simulink model "Linearize_Bare_Airframe"  (R2022a)
settings: Solver=VariableStepAuto  StartTime=0.0  StopTime=10.0  RelTol=1e-3
undefined symbols (not defined in the file): Aactuator, ac, AeroCoeff, EngineTable, F, fs, ft, g, hground, IC, kg, LandingGear, Light, m, MIL, s, Sensor, slug, state0, WMM2020
libraries: aerolibconvert2 x15, simulink x4, aerolibatmos2 x3, aerolibwind2 x3, sharedutil x3, aerolibbdyn x3, aerolibgravity2 x2, sharedtransform x1
(part 1 of 4)
settings Model: Creator=user  LastModifiedBy=user

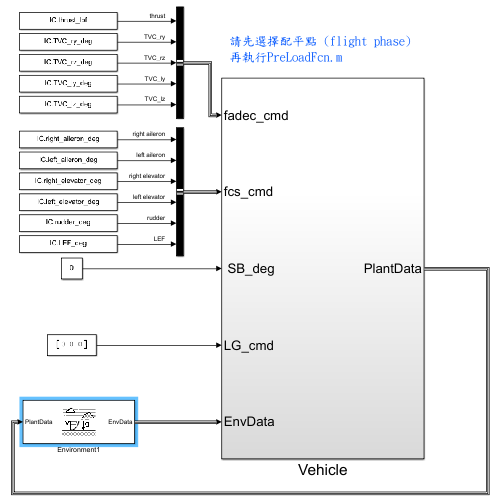
[thumbnail: Simulink's stored preview of the top-level diagram]
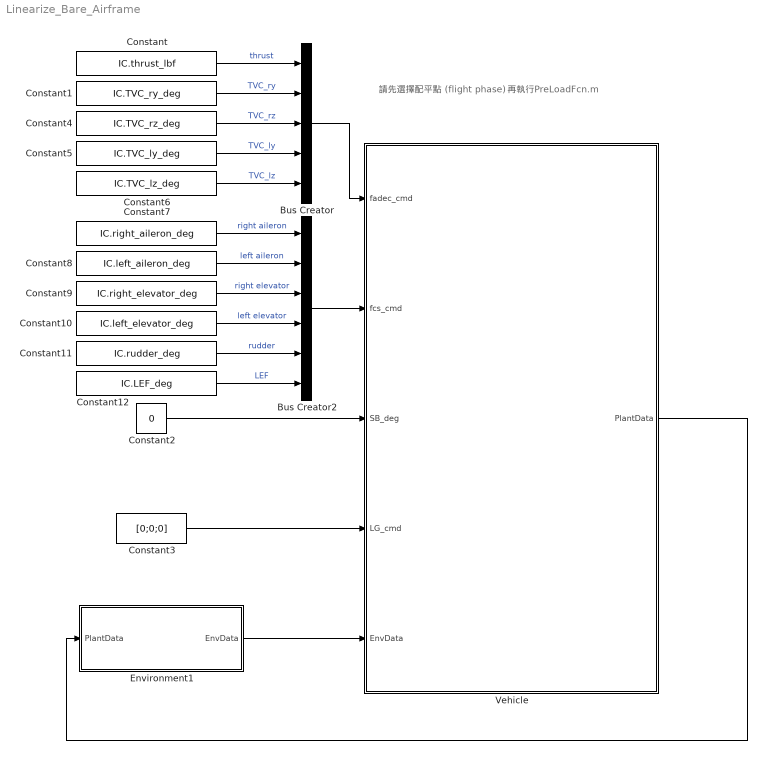
== system Linearize_Bare_Airframe ==
  note: 請先選擇配平點 (flight phase)
      | 再執行PreLoadFcn.m
  Bus Creator : BusCreator  Inputs=5
  Bus Creator2 : BusCreator  Inputs=6
  Constant : Constant  Value=IC.thrust_lbf
  Constant1 : Constant  Value=IC.TVC_ry_deg
  Constant10 : Constant  Value=IC.left_elevator_deg
  Constant11 : Constant  Value=IC.rudder_deg
  Constant12 : Constant  Value=IC.LEF_deg
  Constant2 : Constant  Value=0
  Constant3 : Constant  Value=[0;0;0]
  Constant4 : Constant  Value=IC.TVC_rz_deg
  Constant5 : Constant  Value=IC.TVC_ly_deg
  Constant6 : Constant  Value=IC.TVC_lz_deg
  Constant7 : Constant  Value=IC.right_aileron_deg
  Constant8 : Constant  Value=IC.left_aileron_deg
  Constant9 : Constant  Value=IC.right_elevator_deg
  Environment1 : Subsystem
      mask Display:
      | image('aeroenvironment.bmp','center')
      | % 左側 "Icon transparency" 欄位已選擇 "Opaque with ports"，所以埠名稱會自動顯示，不用再宣告
      | % port_label('input',1,'PlantData')
      | % port_label('output',1,'EnvData')
  Vehicle : Subsystem
  wires:
  Constant3/1 -> Vehicle/4(LG_cmd)
  Constant2/1 -> Vehicle/3(" SB_deg")
  Environment1/1(EnvData) -> Vehicle/5(EnvData)
  Vehicle/1(PlantData) -> Environment1/1(PlantData)
  Constant11/1 -> Bus Creator2/5  "rudder"
  Constant5/1 -> Bus Creator/4  "TVC_ly"
  Constant12/1 -> Bus Creator2/6  "LEF"
  Bus Creator2/1 -> Vehicle/2(fcs_cmd)
  Constant1/1 -> Bus Creator/2  "TVC_ry"
  Constant8/1 -> Bus Creator2/2  "left aileron"
  Constant6/1 -> Bus Creator/5  "TVC_lz"
  Constant/1 -> Bus Creator/1  "thrust"
  Bus Creator/1 -> Vehicle/1(fadec_cmd)
  Constant10/1 -> Bus Creator2/4  "left elevator"
  Constant7/1 -> Bus Creator2/1  "right aileron"
  Constant4/1 -> Bus Creator/3  "TVC_rz"
  Constant9/1 -> Bus Creator2/3  "right elevator"

== system Linearize_Bare_Airframe/Environment1 ==
  note: p, q, r
  note: u, v, w
  note: Wind Models
  note: Atmosphere Model
  note: Altitude must be less than 20000 m (approximately 65620 feet).
  note: 建模注意： EnvData Bus 內要指定公制/英制單位
  note: Magnetic Field
  note: Gravity Model
  note: TODO: 改用這個現成模塊...
      | 但NDI控制器內的重力g是用常數，將產生誤差...
  note: TODO: 改用這個現成模塊...
      | 參考MATLAB Help範例 Quadcopter Project
  note: TODO: 改用現成模塊，改成英制。
      | NDI控制器，不會產生誤差，因為可轉成C程式碼
  note: TODO: 參考MATLAB Help範例 HL-20
      | 將風速效應加到氣動力攻角、側滑角、qbar、Mach、V
  In Bus Element3 : Inport  PortName=PlantData  Element=Vt
  In Bus Element4 : Inport  PortName=PlantData  Element=Vt
  In Bus Element : Inport  PortName=PlantData  Element=DCM_be
  COESA Atmosphere Model : aerolibatmos2/COESA Atmosphere Model  Commented=on  units=English (Velocity in ft/s)  spec=1976 COESA-extended U.S. Standard Atmosphere  model=Profile  profile_var=High temperature  profile_percent=1%  profile_alt=5 km (16404 ft)  envelope_var=High temperature  envelope_percent=1%  action=Warning
  Constant1 : Constant  Value=IC.alt
  Constant12 : Constant  Value=IC.alt
  Constant2 : Constant  Value=IC.Vt
  Density Conversion : aerolibconvert2/Density Conversion  IU=kg/m^3  OU=slug/ft^3
      settings: SourceProductBaseCode=AE
  Discrete Wind Gust Model : aerolibwind2/Discrete Wind Gust Model  Commented=on  units=English (Velocity in ft/s)  Gx=on  Gy=on  Gz=on  t_0=5  d_m=[120 120 80]  v_m=[3.5 3.5 3.0]
  Dryden Wind Turbulence Model (Continuous (+q +r)) : aerolibwind2/Dryden Wind Turbulence Model  (Continuous (+q -r))  Commented=on  units=English (Velocity in ft/s)  spec=MIL-F-8785C  model=Continuous Dryden (+q +r)  W20=15  Wdeg=0  TurbProb=10^-2 - Light  L_high=533.4  Wingspan=10  ts=0.1  Seed=[23341 23342 23343 23344]  T_on=on
  Dynamic Pressure : Subsystem
  Geoid Height : aerolibgravity2/Geoid Height  Commented=on  units=English  gtype=EGM96  datafile='geoidegm96grid'  dtype=double  action=Warning
      settings: AttributesFormatString=EGM2008 Geoid Data Unavailable  SourceProductBaseCode=AE
  ISA Atmosphere Model : aerolibatmos2/ISA Atmosphere Model  Commented=on  custom=off  g=9.80665  gamma=1.4  R=287.0531  L=0.0065  h_trop=11000  h_strat=20000  rho0=1.225  P0=101325  T0=288.15  h0=0
  "ISP " : Subsystem
  Length Conversion : aerolibconvert2/Length Conversion  IU=ft  OU=m
  Mach Number : Subsystem
  Magnetic Field : Constant  Value=[0 0 0]
  Manual Switch : ManualSwitch
  Manual Switch1 : ManualSwitch  CurrentSetting=0
  Pressure Altitude : aerolibatmos2/Pressure Altitude  Commented=on  units=English  action=Warning
      settings: SourceProductBaseCode=AE
  Sum : Sum  Commented=on  Inputs=+++
  Velocity Conversion : aerolibconvert2/Velocity Conversion  IU=m/s  OU=ft/s
  "WGS84 Gravity Model  " : GravityWGS84  Commented=on  units=English
  Wind Shear Model : aerolibwind2/Wind Shear Model  Commented=on  units=English (Velocity in ft/s)  phase=Category C - Terminal Flight Phase  W_20=15  Wdeg=0
  World Magnetic Model : aerolibgravity2/World Magnetic Model  Commented=on  model=WMM2020 (2020-2025)  customFile='WMM2020.COF'  units=English  time_in=on  month=January  day=1  year=2020  action=Error  h_out=off  dec_out=off  inc_out=off  ti_out=off
      settings: SourceProductBaseCode=AE
  gravity (ft/s^2) : Constant  Value=g
  hground (ft) : Constant  Value=hground
  no wind : Constant  Value=[0 0 0]
  no wind1 : Constant  Value=[0 0 0]
  r2d1 : Gain  Commented=on  Gain=-1  SaturateOnIntegerOverflow=on  OutDataTypeStr=Inherit: Same as input  ParamDataTypeStr=Inherit: Same as input
  r2d2 : Gain  Gain=-1  SaturateOnIntegerOverflow=on  OutDataTypeStr=Inherit: Same as input  ParamDataTypeStr=Inherit: Same as input
  Out Bus Element : Outport  PortName=EnvData  Element=Pressure
  Out Bus Element1 : Outport  PortName=EnvData  Element=AirDensity
  Out Bus Element2 : Outport  PortName=EnvData  Element=qbar
  Out Bus Element3 : Outport  PortName=EnvData  Element=Mach
  Out Bus Element4 : Outport  PortName=EnvData  Element=g
  Out Bus Element5 : Outport  PortName=EnvData  Element=hground
  Out Bus Element6 : Outport  PortName=EnvData  Element=MagneticField_NED
  Out Bus Element7 : Outport  PortName=EnvData  Element=AirTemperature_K
  Out Bus Element8 : Outport  PortName=EnvData  Element=SoundSpeed_ms
  Out Bus Element9 : Outport  PortName=EnvData  Element=WindVelocity
  Out Bus Element10 : Outport  PortName=EnvData  Element=WindAngularRates
  wires:
  "ISP "/1(T (K)) -> Out Bus Element7/1
  "ISP "/3(P (HPa)) -> Out Bus Element/1
  "ISP "/4(rho (kg/m^3)) -> Density Conversion/1, Out Bus Element1/1
  hground (ft)/1 -> Out Bus Element5/1
  gravity (ft/s^2)/1 -> Out Bus Element4/1  "Gravity_NED"
  Magnetic Field/1 -> Out Bus Element6/1  "MagneticField_NED"
  Constant12/1 -> r2d2/1
  r2d2/1 -> Length Conversion/1  "h(ft)"
  Length Conversion/1 -> "ISP "/1(h(m))
  "ISP "/2(a (m/s)) -> Out Bus Element8/1, Velocity Conversion/1
  Mach Number/1(Mach) -> Out Bus Element3/1
  Dynamic Pressure/1(qbar) -> Out Bus Element2/1
  Density Conversion/1 -> Dynamic Pressure/2(rho)
  In Bus Element3/1 -> Dynamic Pressure/1(Vt)  "Vt (ft/s)"
  In Bus Element4/1 -> Mach Number/1(Vt)  "Vt (ft/s)"
  Velocity Conversion/1 -> Mach Number/2(a)
  COESA Atmosphere Model/3 -> Pressure Altitude/1
  r2d1/1 -> Dryden Wind Turbulence Model (Continuous (+q +r))/1, Wind Shear Model/1  "h(ft)"
  Constant1/1 -> r2d1/1
  Constant2/1 -> Discrete Wind Gust Model/1, Dryden Wind Turbulence Model (Continuous (+q +r))/2  "Vt (ft/s)"
  In Bus Element/1 -> Wind Shear Model/2, Dryden Wind Turbulence Model (Continuous (+q +r))/3
  Dryden Wind Turbulence Model (Continuous (+q +r))/1 -> Sum/2
  Discrete Wind Gust Model/1 -> Sum/3
  Wind Shear Model/1 -> Sum/1
  Dryden Wind Turbulence Model (Continuous (+q +r))/2 -> Manual Switch1/1  "WindAngularRates"
  Sum/1 -> Manual Switch/2  "WindVelocity"
  Manual Switch/1 -> Out Bus Element9/1
  no wind/1 -> Manual Switch/1
  Manual Switch1/1 -> Out Bus Element10/1
  no wind1/1 -> Manual Switch1/2

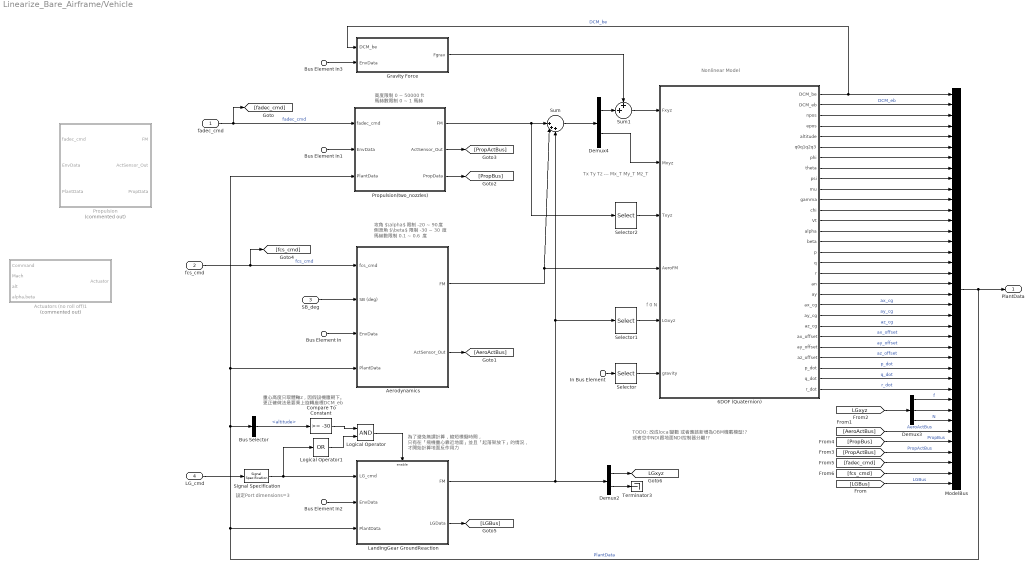
== system Linearize_Bare_Airframe/Vehicle ==
  note: 重心高度只取體軸z，因假設機腹朝下。
      | 更正確做法是要乘上旋轉座標DCM_eb
  note: 為了避免無謂計算，縮短模擬時間，
      | 只有在「飛機重心靠近地面」並且「起落架放下」的情況，
      | 才開始計算地面反作用力
  note: 設定Port dimensions=3
  note: 攻角 $\alpha$ 限制 -20 ~ 90度
      | 側滑角 $\beta$ 限制 -30 ~ 30 度
      | 馬赫數限制 0.1 ~ 0.6 度
  note: Tx
      | Ty
      | Tz
      | ---
      | Mx_T
      | My_T
      | Mz_T
  note: 高度限制 0 ~ 50000 ft
      | 馬赫數限制 0 ~ 1 馬赫
  note: f
      | 0
      | N
  note: TODO: 改成local變數
      | 或者應該新增為OBM機載模型!?
      | 或者空中NDI跟地面NDI控制器分離!?
  note: Nonlinear Model
  fadec_cmd : Inport
  fcs_cmd : Inport  Port=2
  " SB_deg" : Inport  Port=3
  LG_cmd : Inport  Port=4
  Bus Element In{,1..3} (4 alike) : Inport  Port=5  PortName=EnvData
  In Bus Element : Inport  Port=5  PortName=EnvData  Element=g
  6DOF (Quaternion) : Subsystem
  Actuators (no roll off)1 : Subsystem  Commented=on
  Aerodynamics : Subsystem
  Bus Selector : BusSelector  OutputSignals=altitude
  Compare To Constant : simulink/Logic and Bit Operations/Compare To Constant  relop=>=  const=-30  OutDataTypeStr=boolean
  Demux2 : Demux  Outputs=[3, 3]
  Demux3 : Demux  Outputs=3
  Demux4 : Demux  Outputs=[3, 3]
  Gravity Force : Subsystem
  LandingGear GroundReaction : Subsystem
  Logical Operator : Logic  AllPortsSameDT=off  OutDataTypeStr=boolean
  Logical Operator1 : Logic  Operator=OR  Inputs=1  AllPortsSameDT=off  OutDataTypeStr=boolean
  ModelBus : BusCreator  Inputs=38
  Propulsion : Subsystem  Commented=on
  Propulsion(two_nozzles) : Subsystem
  Selector : Selector  InputPortWidth=3  IndexOptions=Index vector (dialog)  Indices=3  OutputSizes=1
  Selector1 : Selector  InputPortWidth=6  IndexOptions=Index vector (dialog)  Indices=[1 2 3]  OutputSizes=1
  Selector2 : Selector  InputPortWidth=6  IndexOptions=Index vector (dialog)  Indices=[1 2 3]  OutputSizes=1
  Signal Specification : SignalSpecification  Dimensions=3
  Sum : Sum  Inputs=||+++
  Sum1 : Sum  Inputs=++|
  Terminator3 : Terminator
  PlantData : Outport
  tag scope: LGxyz=global
  wires:
  " SB_deg"/1 -> Aerodynamics/2(" SB (deg)")
  Aerodynamics/1(FM) -> Sum/2, 6DOF (Quaternion)/4(AeroFM)
  Aerodynamics/2(ActSensor_Out) -> [AeroActBus]
  Propulsion(two_nozzles)/1(FM) -> Selector2/1, Sum/1
  fcs_cmd/1 -> Aerodynamics/1(fcs_cmd), [fcs_cmd]  "fcs_cmd"
  fadec_cmd/1 -> Propulsion(two_nozzles)/1(fadec_cmd), [fadec_cmd]  "fadec_cmd"
  Propulsion(two_nozzles)/2(ActSensor_Out) -> [PropActBus]
  Propulsion(two_nozzles)/3(PropData) -> [PropBus]
  Sum/1 -> Demux4/1
  Sum1/1 -> 6DOF (Quaternion)/1(Fxyz)
  Bus Element In/1 -> Aerodynamics/3(EnvData)
  Bus Element In1/1 -> Propulsion(two_nozzles)/2(EnvData)
  LandingGear GroundReaction/1(FM) -> Demux2/1, Sum/3, Selector1/1
  Selector1/1 -> 6DOF (Quaternion)/5(LGxyz)
  Demux2/1 -> [LGxyz]
  Demux2/2 -> Terminator3/1
  Signal Specification/1 -> Logical Operator1/1, LandingGear GroundReaction/1(LG_cmd)
  LandingGear GroundReaction/2(LGData) -> [LGBus]
  Logical Operator/1 -> LandingGear GroundReaction/Enable
  Compare To Constant/1 -> Logical Operator/1
  Bus Selector/1 -> Compare To Constant/1  "<altitude>"
  Logical Operator1/1 -> Logical Operator/2
  LG_cmd/1 -> Signal Specification/1
  Gravity Force/1(Fgrav) -> Sum1/1
  Demux4/1 -> Sum1/2
  Bus Element In3/1 -> Gravity Force/2(EnvData)
  Bus Element In2/1 -> LandingGear GroundReaction/2(EnvData)
  In Bus Element/1 -> Selector/1
  [PropActBus] -> ModelBus/35  "PropActBus"
  Demux3/2 -> ModelBus/31
  6DOF (Quaternion)/22(ay_cg) -> ModelBus/22  "ay_cg"
  Demux3/3 -> ModelBus/32  "N"
  Demux3/1 -> ModelBus/30  "f"
  6DOF (Quaternion)/2(DCM_eb) -> ModelBus/2  "DCM_eb"
  6DOF (Quaternion)/18(r) -> ModelBus/18
  6DOF (Quaternion)/8(theta) -> ModelBus/8
  [fadec_cmd] -> ModelBus/36
  6DOF (Quaternion)/21(ax_cg) -> ModelBus/21  "ax_cg"
  [LGBus] -> ModelBus/38  "LGBus"
  6DOF (Quaternion)/3(npos) -> ModelBus/3
  6DOF (Quaternion)/10(mu) -> ModelBus/10
  [fcs_cmd] -> ModelBus/37
  [AeroActBus] -> ModelBus/33  "AeroActBus"
  6DOF (Quaternion)/16(p) -> ModelBus/16
  6DOF (Quaternion)/17(q) -> ModelBus/17
  6DOF (Quaternion)/13(Vt) -> ModelBus/13
  6DOF (Quaternion)/29(r_dot) -> ModelBus/29  "r_dot"
  6DOF (Quaternion)/24(ax_offset) -> ModelBus/24  "ax_offset"
  6DOF (Quaternion)/28(q_dot) -> ModelBus/28  "q_dot"
  6DOF (Quaternion)/19(an) -> ModelBus/19
  6DOF (Quaternion)/20(ay) -> ModelBus/20
  6DOF (Quaternion)/6(q0q1q2q3) -> ModelBus/6
  6DOF (Quaternion)/11(gamma) -> ModelBus/11
  6DOF (Quaternion)/27(p_dot) -> ModelBus/27  "p_dot"
  6DOF (Quaternion)/9(psi) -> ModelBus/9
  6DOF (Quaternion)/5(altitude) -> ModelBus/5
  6DOF (Quaternion)/7(phi) -> ModelBus/7
  6DOF (Quaternion)/14(alpha) -> ModelBus/14
  6DOF (Quaternion)/4(epos) -> ModelBus/4
  6DOF (Quaternion)/15(beta) -> ModelBus/15
  6DOF (Quaternion)/1(DCM_be) -> Gravity Force/1(DCM_be), ModelBus/1  "DCM_be"
  6DOF (Quaternion)/23(az_cg) -> ModelBus/23  "az_cg"
  [LGxyz] -> Demux3/1
  ModelBus/1 -> PlantData/1, LandingGear GroundReaction/3(PlantData), Bus Selector/1, Propulsion(two_nozzles)/3(PlantData), Aerodynamics/4(PlantData)  "PlantData"
  6DOF (Quaternion)/25(ay_offset) -> ModelBus/25  "ay_offset"
  6DOF (Quaternion)/12(chi) -> ModelBus/12
  [PropBus] -> ModelBus/34  "PropBus"
  6DOF (Quaternion)/26(az_offset) -> ModelBus/26  "az_offset"
  Demux4/2 -> 6DOF (Quaternion)/2(Mxyz)
  Selector2/1 -> 6DOF (Quaternion)/3(Txyz)
  Selector/1 -> 6DOF (Quaternion)/6(gravity)

== system Linearize_Bare_Airframe/Environment1/Dynamic Pressure ==
  Vt : Inport
  rho : Inport  Port=2
  1/2rhoV^2 : Gain  Gain=1/2  SaturateOnIntegerOverflow=on  OutDataTypeStr=Inherit: Same as input  ParamDataTypeStr=Inherit: Same as input
  Product2 : Product  InputSameDT=on  SaturateOnIntegerOverflow=on  OutDataTypeStr=Inherit: Same as first input
  Square : Math  Operator=square  SignedPower=on
  qbar : Outport
  wires:
  rho/1 -> Product2/2
  Square/1 -> Product2/1
  1/2rhoV^2/1 -> qbar/1
  Product2/1 -> 1/2rhoV^2/1
  Vt/1 -> Square/1

== system Linearize_Bare_Airframe/Environment1/ISP  ==
  note: 1 T
      | 2 a (Speed of sound)
      | 3 P
      | 4 rho
      | 5 g
      | 6 mu (Coefficient of viscosity)
  h(m) : Inport
  Demux : Demux  Outputs=[1,1,1,1,1,1]
      settings: DisplayOption=none
  MATLAB Function : MATLAB Function  TreatAsAtomicUnit=on
  end8 : Terminator
  end9 : Terminator
  T (K) : Outport  VectorParamsAs1DForOutWhenUnconnected=off
  a (m/s) : Outport  Port=2  VectorParamsAs1DForOutWhenUnconnected=off
  P (HPa) : Outport  Port=3  VectorParamsAs1DForOutWhenUnconnected=off
  rho (kg/m^3) : Outport  Port=4  VectorParamsAs1DForOutWhenUnconnected=off
  wires:
  MATLAB Function/1(ISP_output) -> Demux/1
  h(m)/1 -> MATLAB Function/1(h)
  Demux/4 -> rho (kg/m^3)/1  "rho(kg/m^3)"
  Demux/2 -> a (m/s)/1  "a(m/s)"
  Demux/1 -> T (K)/1  "T(K)"
  Demux/5 -> end8/1  "g (m/s^2)"
  Demux/6 -> end9/1  "mu"
  Demux/3 -> P (HPa)/1  "P(Pa)"

== system Linearize_Bare_Airframe/Environment1/Mach Number ==
  Vt : Inport
  a : Inport  Port=2
  Product1 : Product  Inputs=*/  InputSameDT=on  SaturateOnIntegerOverflow=on  OutDataTypeStr=Inherit: Same as first input
  Mach : Outport  Unit=1  VectorParamsAs1DForOutWhenUnconnected=off
  wires:
  Vt/1 -> Product1/1
  a/1 -> Product1/2
  Product1/1 -> Mach/1

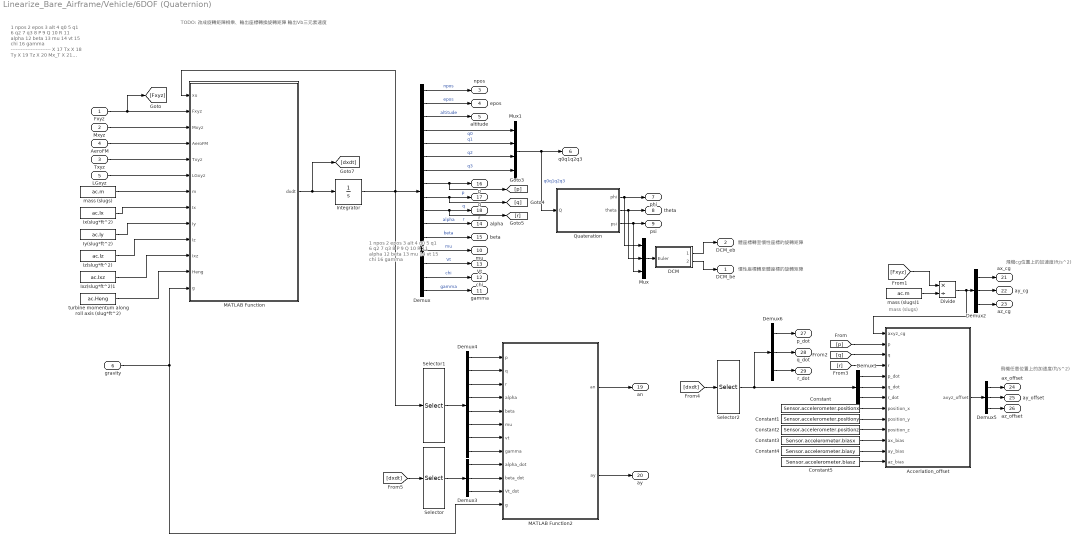
== system Linearize_Bare_Airframe/Vehicle/6DOF (Quaternion) ==
  note: TODO: 改成旋轉矩陣相乘、輸出座標轉換旋轉矩陣
      | 輸出Vb三元素速度
  note: 1 npos
      | 2 epos
      | 3 alt
      | 4 q0
      | 5 q1
      | 6 q2
      | 7 q3
      | 8 P
      | 9 Q
      | 10 R
      | 11 alpha
      | 12 beta
      | 13 mu
      | 14 vt
      | 15 chi
      | 16 gamma
      | ------------------------
      | X 17 Tx
      | X 18 Ty
      | X 19 Tz
      | X 20 Mx_T
      | X 21 My_T
      | X 22 Mz_T
      | X 23 T
      | --------------------
      | X 24 ele
      | X 25 ail
      | X 26 rud
      | -------------------
      | X 27 delta_z
      | X 28 delta_y
      | -----------------
      | X 29 qbar
      | -----------------
      | X 30 CXT
      | X 31 CYT
      | X 32 CZT
      | X 33 CLT
      | X 34 CMT
      | X 35 CNT
      | -----------------
      | X 36 lef
  note: 1 npos
      | 2 epos
      | 3 alt
      | 4 q0
      | 5 q1
      | 6 q2
      | 7 q3
      | 8 P
      | 9 Q
      | 10 R
      | 11 alpha
      | 12 beta
      | 13 mu
      | 14 vt
      | 15 chi
      | 16 gamma
  note: 慣性座標轉至體座標的旋轉矩陣
  note: 體座標轉至慣性座標的旋轉矩陣
  note: mass (slugs)
  note: 飛機cg位置上的加速度(ft/s^2)
  note: 飛機任意位置上的加速度(ft/s^2)
  Fxyz : Inport
  Mxyz : Inport  Port=2
  Txyz : Inport  Port=3
  AeroFM : Inport  Port=4
  LGxyz : Inport  Port=5
  gravity : Inport  Port=6
  Accerlation_offset : Subsystem
  Constant : Constant  Value=Sensor.accelerometer.positionx
  Constant1 : Constant  Value=Sensor.accelerometer.positiony
  Constant2 : Constant  Value=Sensor.accelerometer.positionz
  Constant3 : Constant  Value=Sensor.accelerometer.biasx
  Constant4 : Constant  Value=Sensor.accelerometer.biasy
  Constant5 : Constant  Value=Sensor.accelerometer.biasz
  DCM : Subsystem
  Demux : Demux  Outputs=16
      settings: DisplayOption=none
  Demux{1..3,5..6} (5 alike) : Demux  Outputs=3
  Demux4 : Demux  Outputs=8
  Divide : Product  Inputs=*/
  Integrator : Integrator  InitialCondition=state0  ContinuousStateAttributes={'npos', 'epos', 'alt', 'q0', 'q1', 'q2', 'q3', 'P', 'Q', 'R', 'alpha', 'beta', 'mu', 'vt', 'chi', 'gamma'}
  Ix(slug*ft^2) : Constant  Value=ac.Ix
  Ixz(slug*ft^2)1 : Constant  Value=ac.Ixz
  Iy(slug*ft^2) : Constant  Value=ac.Iy
  Iz(slug*ft^2) : Constant  Value=ac.Iz
  MATLAB Function : MATLAB Function  TreatAsAtomicUnit=on
  MATLAB Function2 : MATLAB Function  TreatAsAtomicUnit=on
  Mux : Mux  Inputs=3
  Mux1 : Mux  Inputs=[1,1,1,1]
  Quateration : MATLAB Function  TreatAsAtomicUnit=on
  Selector : Selector  InputPortWidth=16  IndexOptions=Index vector (dialog)  Indices=[11 12 14]  OutputSizes=3
  Selector1 : Selector  InputPortWidth=16  IndexOptions=Index vector (dialog)  Indices=[8:14 16]  OutputSizes=3
  Selector2 : Selector  InputPortWidth=16  IndexOptions=Index vector (dialog)  Indices=[8 9 10]  OutputSizes=3
  mass (slugs) : Constant  Value=ac.m
  mass (slugs)1 : Constant  Value=ac.m
  turbine momentum along roll axis (slug*ft^2) : Constant  Value=ac.Heng
  DCM_be : Outport
  DCM_eb : Outport  Port=2
  npos : Outport  Port=3  VectorParamsAs1DForOutWhenUnconnected=off
  epos : Outport  Port=4  VectorParamsAs1DForOutWhenUnconnected=off
  altitude : Outport  Port=5  VectorParamsAs1DForOutWhenUnconnected=off
  q0q1q2q3 : Outport  Port=6
  phi : Outport  Port=7  VectorParamsAs1DForOutWhenUnconnected=off
  theta : Outport  Port=8  VectorParamsAs1DForOutWhenUnconnected=off
  psi : Outport  Port=9  VectorParamsAs1DForOutWhenUnconnected=off
  mu : Outport  Port=10  VectorParamsAs1DForOutWhenUnconnected=off
  gamma : Outport  Port=11  VectorParamsAs1DForOutWhenUnconnected=off
  chi : Outport  Port=12  VectorParamsAs1DForOutWhenUnconnected=off
  Vt : Outport  Port=13  VectorParamsAs1DForOutWhenUnconnected=off
  alpha : Outport  Port=14  VectorParamsAs1DForOutWhenUnconnected=off
  beta : Outport  Port=15  VectorParamsAs1DForOutWhenUnconnected=off
  p : Outport  Port=16  VectorParamsAs1DForOutWhenUnconnected=off
  q : Outport  Port=17  VectorParamsAs1DForOutWhenUnconnected=off
  r : Outport  Port=18  VectorParamsAs1DForOutWhenUnconnected=off
  an : Outport  Port=19
  ay : Outport  Port=20
  ax_cg : Outport  Port=21
  ay_cg : Outport  Port=22
  az_cg : Outport  Port=23
  ax_offset : Outport  Port=24
  ay_offset : Outport  Port=25
  az_offset : Outport  Port=26
  p_dot : Outport  Port=27
  q_dot : Outport  Port=28
  r_dot : Outport  Port=29
  wires:
  Demux/2 -> epos/1  "epos"
  Demux/3 -> altitude/1  "altitude"
  Integrator/1 -> MATLAB Function/1(xu), Demux/1, Selector1/1
  Demux/1 -> npos/1  "npos"
  Demux/5 -> Mux1/2  "q1"
  Demux/4 -> Mux1/1  "q0"
  Demux/7 -> Mux1/4  "q3"
  Demux/6 -> Mux1/3  "q2"
  Demux/8 -> p/1, [p]  "p"
  Demux/9 -> q/1, [q]  "q"
  Demux/10 -> r/1, [r]  "r"
  Demux/11 -> alpha/1  "alpha"
  Demux/12 -> beta/1  "beta"
  Demux/13 -> mu/1  "mu"
  Demux/14 -> Vt/1  "Vt"
  Demux/15 -> chi/1  "chi"
  Demux/16 -> gamma/1  "gamma"
  Mux1/1 -> q0q1q2q3/1, Quateration/1(Q)  "q0q1q2q3"
  AeroFM/1 -> MATLAB Function/4(AeroFM)
  Mxyz/1 -> MATLAB Function/3(Mxyz)
  Fxyz/1 -> [Fxyz], MATLAB Function/2(Fxyz)
  Txyz/1 -> MATLAB Function/5(Txyz)
  gravity/1 -> MATLAB Function2/12(g), MATLAB Function/13(g)
  Ix(slug*ft^2)/1 -> MATLAB Function/8(Ix)
  Iy(slug*ft^2)/1 -> MATLAB Function/9(Iy)
  Iz(slug*ft^2)/1 -> MATLAB Function/10(Iz)
  Ixz(slug*ft^2)1/1 -> MATLAB Function/11(Ixz)
  turbine momentum along roll axis (slug*ft^2)/1 -> MATLAB Function/12(Heng)
  mass (slugs)/1 -> MATLAB Function/7(m)
  Selector/1 -> Demux3/1
  Demux3/1 -> MATLAB Function2/9(alpha_dot)
  Demux3/2 -> MATLAB Function2/10(beta_dot)
  Demux3/3 -> MATLAB Function2/11(Vt_dot)
  Selector1/1 -> Demux4/1
  Demux4/1 -> MATLAB Function2/1(p)
  Demux4/2 -> MATLAB Function2/2(q)
  Demux4/3 -> MATLAB Function2/3(r)
  Demux4/4 -> MATLAB Function2/4(alpha)
  Demux4/5 -> MATLAB Function2/5(beta)
  Demux4/6 -> MATLAB Function2/6(mu)
  Demux4/7 -> MATLAB Function2/7(vt)
  Demux4/8 -> MATLAB Function2/8(gamma)
  MATLAB Function2/1(an) -> an/1
  MATLAB Function2/2(ay) -> ay/1
  LGxyz/1 -> MATLAB Function/6(LGxyz)
  Quateration/3(psi) -> Mux/3, psi/1
  Quateration/2(theta) -> theta/1, Mux/2
  Quateration/1(phi) -> phi/1, Mux/1
  Mux/1 -> DCM/1(Euler)
  DCM/1(DCM_eb) -> DCM_eb/1
  DCM/2(DCM_be) -> DCM_be/1
  Constant4/1 -> Accerlation_offset/12(ay_bias)
  Accerlation_offset/1(axyz_offset) -> Demux5/1
  Constant/1 -> Accerlation_offset/8(position_x)
  Selector2/1 -> Demux6/1, Demux1/1
  Demux6/1 -> p_dot/1
  Demux1/2 -> Accerlation_offset/6(q_dot)
  Demux6/2 -> q_dot/1
  Demux5/1 -> ax_offset/1
  Demux5/3 -> az_offset/1
  Demux6/3 -> r_dot/1
  [dxdt] -> Selector2/1
  Demux2/1 -> ax_cg/1
  mass (slugs)1/1 -> Divide/2
  Demux1/1 -> Accerlation_offset/5(p_dot)
  Demux1/3 -> Accerlation_offset/7(r_dot)
  [p] -> Accerlation_offset/2(p)
  [Fxyz] -> Divide/1
  [q] -> Accerlation_offset/3(q)
  Constant1/1 -> Accerlation_offset/9(position_y)
  [r] -> Accerlation_offset/4(r)
  Constant3/1 -> Accerlation_offset/11(ax_bias)
  Constant5/1 -> Accerlation_offset/13(az_bias)
  Demux2/3 -> az_cg/1
  Divide/1 -> Accerlation_offset/1(axyz_cg), Demux2/1
  Constant2/1 -> Accerlation_offset/10(position_z)
  Demux5/2 -> ay_offset/1
  Demux2/2 -> ay_cg/1
  MATLAB Function/1(dxdt) -> [dxdt], Integrator/1
  [dxdt] -> Selector/1

== system Linearize_Bare_Airframe/Vehicle/Actuators (no roll off)1 ==
  note: 這種建模方式會得到跟順淵不同的結果
  Command : Inport
  "Mach " : Inport  Port=2
  alt : Inport  Port=3
  alpha,beta : Inport  Port=4
  Aileron Saturation : Saturate  UpperLimit=21.5  LowerLimit=-21.5
  Demux1 : Demux  Outputs=6
  Elevator Saturation : Saturate  UpperLimit=25  LowerLimit=-25
  Engine block : Subsystem
  Fcn : Fcn  Expr=u(1)*cos(u(2))*cos(u(3))
  Integrator (degrees) : Integrator  Commented=through  InitialCondition=0.015206  UpperSaturationLimit=30  LowerSaturationLimit=-30
  Integrator (degrees)1 : Integrator  Commented=through  UpperSaturationLimit=30  LowerSaturationLimit=-30
  Integrator (degrees)2 : Integrator  Commented=on  UpperSaturationLimit=30  LowerSaturationLimit=-30
  Integrator(degrees) : Integrator  Commented=on  InitialCondition=-0.051516  UpperSaturationLimit=21.5  LowerSaturationLimit=-21.5
  "Integrator(degrees) " : Integrator  Commented=on  InitialCondition=-4.2454  UpperSaturationLimit=25  LowerSaturationLimit=-25
  Mux1 : Mux  Inputs=2
  Mux9 : Mux  Inputs=6
  Rate Limiter : RateLimiter  RisingSlewLimit=+60  FallingSlewLimit=-60  SampleTimeMode=inherited
  Rate Limiter1 : RateLimiter  RisingSlewLimit=+80  FallingSlewLimit=-80  SampleTimeMode=inherited
  Rate Limiter2 : RateLimiter  RisingSlewLimit=+120  FallingSlewLimit=-120  SampleTimeMode=inherited
  Rate Limiter3 : RateLimiter  RisingSlewLimit=+60  FallingSlewLimit=-60  SampleTimeMode=inherited
  Rate Limiter4 : RateLimiter  RisingSlewLimit=+60  FallingSlewLimit=-60  SampleTimeMode=inherited
  Rudder Saturation : Saturate  UpperLimit=30  LowerLimit=-30
  Saturation : Saturate  UpperLimit=50000  LowerLimit=0
  Saturation Dynamic : simulink/Discontinuities/Saturation Dynamic  OutMin=[]  OutMax=[]  OutDataTypeStr=Inherit: Same as second input  OutDataType=fixdt(1, 16)  OutScaling=2^-10  DoSatur=off
  TVC_Y Saturation : Saturate  UpperLimit=15  LowerLimit=-15
  TVC_Z Saturation : Saturate  UpperLimit=15  LowerLimit=-15
  Transfer Fcn{,1..4} (5 alike) : TransferFcn  Numerator=[20.202]  Denominator=[1 20.202]
  r2d2 : Gain  Gain=-1  SaturateOnIntegerOverflow=on  OutDataTypeStr=Inherit: Same as input  ParamDataTypeStr=Inherit: Same as input
  Actuator : Outport  VectorParamsAs1DForOutWhenUnconnected=off
  wires:
  Mux9/1 -> Actuator/1
  Command/1 -> Demux1/1
  Transfer Fcn/1 -> Mux9/2  "elevator"
  Transfer Fcn1/1 -> Mux9/3  "Aileron"
  Transfer Fcn2/1 -> Mux9/4  "Rudder"
  Saturation Dynamic/1 -> Mux9/1  "thrust"
  Transfer Fcn4/1 -> Mux9/6  "yaw vector"
  Transfer Fcn3/1 -> Mux9/5  "pitch vector"
  r2d2/1 -> Saturation/1
  alt/1 -> r2d2/1
  Demux1/1 -> Saturation Dynamic/2
  "Mach "/1 -> Mux1/1
  alpha,beta/1 -> Mux1/2
  Mux1/1 -> Fcn/1
  Fcn/1 -> Engine block/1(Mach)
  Saturation/1 -> Engine block/2(Attitude)
  Engine block/2(T_min) -> Saturation Dynamic/3
  Engine block/1(T_max) -> Saturation Dynamic/1
  Demux1/2 -> Elevator Saturation/1
  Elevator Saturation/1 -> Rate Limiter/1
  Demux1/3 -> Aileron Saturation/1
  Aileron Saturation/1 -> Rate Limiter1/1
  Demux1/4 -> Rudder Saturation/1
  Rudder Saturation/1 -> Rate Limiter2/1
  Demux1/5 -> TVC_Z Saturation/1
  TVC_Z Saturation/1 -> Rate Limiter3/1
  Demux1/6 -> TVC_Y Saturation/1
  TVC_Y Saturation/1 -> Rate Limiter4/1
  Rate Limiter/1 -> Transfer Fcn/1
  Rate Limiter1/1 -> Transfer Fcn1/1
  Rate Limiter2/1 -> Transfer Fcn2/1
  Rate Limiter3/1 -> Transfer Fcn3/1
  Rate Limiter4/1 -> Transfer Fcn4/1

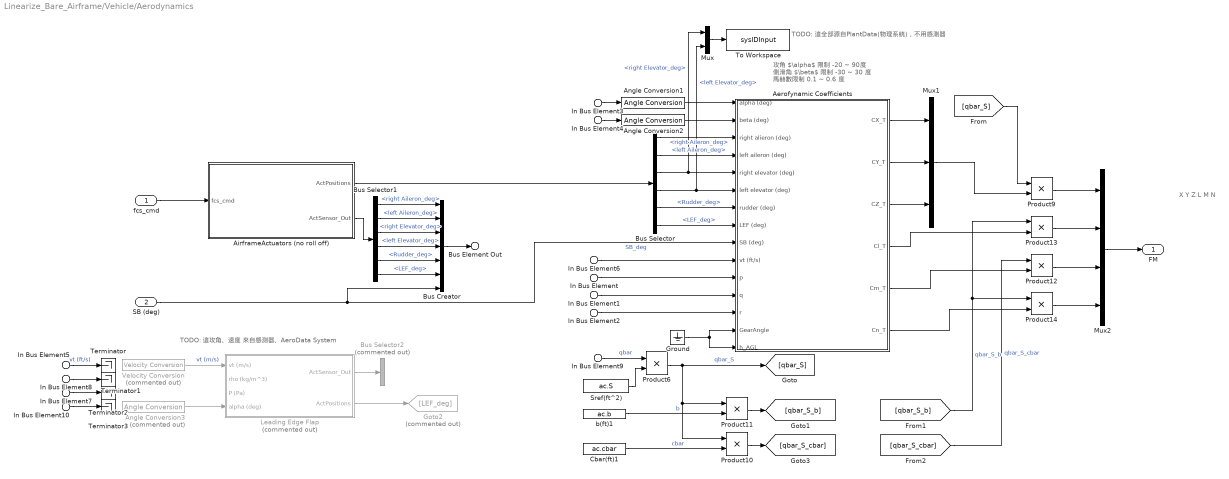
== system Linearize_Bare_Airframe/Vehicle/Aerodynamics ==
  note: TODO: 這全部源自PlantData(物理系統)，不用感測器
  note: TODO: 這攻角、速度 來自感測器、AeroData System
  note: X
      | Y
      | Z
      | L
      | M
      | N
  note: 攻角 $\alpha$ 限制 -20 ~ 90度
      | 側滑角 $\beta$ 限制 -30 ~ 30 度
      | 馬赫數限制 0.1 ~ 0.6 度
  fcs_cmd : Inport
  " SB (deg)" : Inport  Port=2
  In Bus Element7 : Inport  Port=3  PortName=EnvData  Element=Pressure
  In Bus Element8 : Inport  Port=3  PortName=EnvData  Element=AirDensity
  In Bus Element9 : Inport  Port=3  PortName=EnvData  Element=qbar
  In Bus Element : Inport  Port=4  PortName=PlantData  Element=p
  In Bus Element1 : Inport  Port=4  PortName=PlantData  Element=q
  In Bus Element2 : Inport  Port=4  PortName=PlantData  Element=r
  In Bus Element3 : Inport  Port=4  PortName=PlantData  Element=alpha
  In Bus Element10 : Inport  Port=4  PortName=PlantData  Element=alpha
  In Bus Element4 : Inport  Port=4  PortName=PlantData  Element=beta
  In Bus Element6 : Inport  Port=4  PortName=PlantData  Element=Vt
  In Bus Element5 : Inport  Port=4  PortName=PlantData  Element=Vt
  Aerofynamic Coefficients : Subsystem
  AirframeActuators (no roll off) : Subsystem
  Angle Conversion1 : aerolibconvert2/Angle Conversion  IU=rad  OU=deg
  Angle Conversion2 : aerolibconvert2/Angle Conversion  IU=rad  OU=deg
  Angle Conversion3 : aerolibconvert2/Angle Conversion  Commented=on  IU=rad  OU=deg
  Bus Creator : BusCreator  Inputs=7
  Bus Selector : BusSelector  OutputSignals=right Aileron_deg,left Aileron_deg,right Elevator_deg,left Elevator_deg,Rudder_deg,LEF_deg
  Bus Selector1 : BusSelector  OutputSignals=right Aileron_deg,left Aileron_deg,right Elevator_deg,left Elevator_deg,Rudder_deg,LEF_deg
  Bus Selector2 : BusSelector  Commented=on  OutputSignals=LEF_deg
  Cbar(ft)1 : Constant  Value=ac.cbar
  Goto2 : Goto  Commented=on  GotoTag=LEF_deg
  Ground : Ground
  Leading Edge Flap : Subsystem  Commented=on
  Mux : Mux  Inputs=2
  Mux1 : Mux  Inputs=3
  Mux2 : Mux
  Product{6,9..14} (7 alike) : Product
  Sref(ft^2) : Constant  Value=ac.S
  Terminator{,1..3} (4 alike) : Terminator
  To Workspace : ToWorkspace  VariableName=sysIDInput  SaveFormat=Timeseries  SampleTime=1/fs
  Velocity Conversion : aerolibconvert2/Velocity Conversion  Commented=on  IU=ft/s  OU=m/s
  b(ft)1 : Constant  Value=ac.b
  FM : Outport
  Bus Element Out : Outport  Port=2  PortName=ActSensor_Out
  wires:
  " SB (deg)"/1 -> Aerofynamic Coefficients/9(SB (deg)), Bus Creator/7  "SB_deg"
  In Bus Element1/1 -> Aerofynamic Coefficients/12(q)
  In Bus Element/1 -> Aerofynamic Coefficients/11(p)
  Angle Conversion2/1 -> Aerofynamic Coefficients/2(beta (deg))
  Angle Conversion1/1 -> Aerofynamic Coefficients/1(alpha (deg))
  In Bus Element2/1 -> Aerofynamic Coefficients/13(r)
  Ground/1 -> Aerofynamic Coefficients/15(h_AGL), Aerofynamic Coefficients/14(GearAngle)
  Mux1/1 -> Product9/2
  [qbar_S] -> Product9/1
  Aerofynamic Coefficients/6(Cn_T) -> Product14/2
  Aerofynamic Coefficients/5(Cm_T) -> Product12/2
  [qbar_S_cbar] -> Product12/1  "qbar_S_cbar"
  Aerofynamic Coefficients/4(Cl_T) -> Product13/2
  [qbar_S_b] -> Product13/1, Product14/1  "qbar_S_b"
  Aerofynamic Coefficients/1(CX_T) -> Mux1/1
  Aerofynamic Coefficients/2(CY_T) -> Mux1/2
  Aerofynamic Coefficients/3(CZ_T) -> Mux1/3
  Product13/1 -> Mux2/2
  Product12/1 -> Mux2/3
  Product14/1 -> Mux2/4
  Product9/1 -> Mux2/1
  Mux2/1 -> FM/1
  Sref(ft^2)/1 -> Product6/2
  b(ft)1/1 -> Product11/2  "b"
  Product11/1 -> [qbar_S_b]
  Product10/1 -> [qbar_S_cbar]
  Cbar(ft)1/1 -> Product10/2  "cbar"
  In Bus Element9/1 -> Product6/1  "qbar"
  Product6/1 -> Product11/1, Product10/1, [qbar_S]  "qbar_S"
  Leading Edge Flap/2(ActPositions) -> Goto2/1
  Velocity Conversion/1 -> Leading Edge Flap/1(vt (m/s))  "vt (m/s)"
  In Bus Element6/1 -> Aerofynamic Coefficients/10(vt (ft/s))
  In Bus Element8/1 -> Terminator1/1
  In Bus Element7/1 -> Terminator2/1
  AirframeActuators (no roll off)/1(ActPositions) -> Bus Selector/1
  fcs_cmd/1 -> AirframeActuators (no roll off)/1(fcs_cmd)
  In Bus Element3/1 -> Angle Conversion1/1
  In Bus Element4/1 -> Angle Conversion2/1
  In Bus Element5/1 -> Terminator/1  "vt (ft/s)"
  AirframeActuators (no roll off)/2(ActSensor_Out) -> Bus Selector1/1
  Bus Creator/1 -> Bus Element Out/1
  In Bus Element10/1 -> Terminator3/1
  Angle Conversion3/1 -> Leading Edge Flap/4(alpha (deg))
  Leading Edge Flap/1(ActSensor_Out) -> Bus Selector2/1
  Bus Selector1/1 -> Bus Creator/1  "<right Aileron_deg>"
  Bus Selector1/2 -> Bus Creator/2  "<left Aileron_deg>"
  Bus Selector1/3 -> Bus Creator/3  "<right Elevator_deg>"
  Bus Selector1/4 -> Bus Creator/4  "<left Elevator_deg>"
  Bus Selector1/5 -> Bus Creator/5  "<Rudder_deg>"
  Bus Selector1/6 -> Bus Creator/6  "<LEF_deg>"
  Bus Selector/1 -> Aerofynamic Coefficients/3(right alieron (deg))  "<right Aileron_deg>"
  Bus Selector/2 -> Aerofynamic Coefficients/4(left aileron (deg))  "<left Aileron_deg>"
  Bus Selector/3 -> Mux/1, Aerofynamic Coefficients/5(right elevator (deg))  "<right Elevator_deg>"
  Bus Selector/4 -> Mux/2, Aerofynamic Coefficients/6(left elevator (deg))  "<left Elevator_deg>"
  Bus Selector/5 -> Aerofynamic Coefficients/7(rudder (deg))  "<Rudder_deg>"
  Bus Selector/6 -> Aerofynamic Coefficients/8(LEF (deg))  "<LEF_deg>"
  Mux/1 -> To Workspace/1

== system Linearize_Bare_Airframe/Vehicle/Gravity Force ==
  note: 轉成行向量(column vector)
  note: 註：重力不會對飛機產生力矩，
      | 因為重力永遠作用在飛機重心上，
      | 力臂=0，所以力矩=0
  DCM_be : Inport
  In Bus Element : Inport  Port=2  PortName=EnvData  Element=g
  Gravity in Earth Axis : Gain  Gain=ac.m
  Reshape : Reshape  OutputDimensionality=Column vector (2-D)
  To Body Axes : Product  Multiplication=Matrix(*)
  Fgrav : Outport
  wires:
  In Bus Element/1 -> Gravity in Earth Axis/1
  To Body Axes/1 -> Fgrav/1
  DCM_be/1 -> To Body Axes/1
  Gravity in Earth Axis/1 -> Reshape/1
  Reshape/1 -> To Body Axes/2

== system Linearize_Bare_Airframe/Vehicle/LandingGear GroundReaction ==
  note: 定義：
      | 慣性座標+Z軸朝上
      | 體座標+Z軸朝下
  note: 詹庭宇:
      | 此起落架模組源自MATLAB Simulink Example:HL-20
      | 我有做
      | 1.正負號的訂正
      | 2.拿掉/忽略輪胎側向力
  note: 詹庭宇:拿掉/忽略輪胎側向力模型，Fy=0
  LG_cmd : Inport
  In Bus Element4 : Inport  Port=2  PortName=EnvData  Element=hground
  In Bus Element5 : Inport  Port=2  PortName=EnvData  Element=hground
  In Bus Element6 : Inport  Port=2  PortName=EnvData  Element=hground
  In Bus Element3 : Inport  Port=3  PortName=PlantData
  In Bus Element1 : Inport  Port=3  PortName=PlantData
  In Bus Element2 : Inport  Port=3  PortName=PlantData
  Enable : EnablePort
  Demux : Demux  Outputs=3
  L Main Gear Geometry Forces and Moments : Subsystem  TreatAsAtomicUnit=on
  LeftMain : Selector  NumberOfDimensions=2  InputPortWidth=3  IndexOptions=Select all,Index vector (dialog)  Indices=-1,1  OutputSizes=1
  Nose : Selector  NumberOfDimensions=2  InputPortWidth=3  IndexOptions=Select all,Index vector (dialog)  Indices=-1,3  OutputSizes=1
  Nose Gear Geometry Forces and Moments : Subsystem  TreatAsAtomicUnit=on
  Pos_full_extend_ft Rows are X,Y,Z;cols are Left,Right,Nose gear Measured from CG in fts : Constant  Value=[-1.8405,-1.8405,9.9132 ; -3.8753,3.8753,0 ; 5.9161,5.9161, 6.2905]
  R Main Gear Geometry Forces and Moments : Subsystem  TreatAsAtomicUnit=on
  RightMain : Selector  NumberOfDimensions=2  InputPortWidth=3  IndexOptions=Select all,Index vector (dialog)  Indices=-1,2  OutputSizes=1
  Sum2 : Sum  Inputs=+++  InputSameDT=on  SaturateOnIntegerOverflow=on  OutDataTypeStr=Inherit: Same as first input
  FM : Outport
  Out Bus Element3 : Outport  Port=2  VectorParamsAs1DForOutWhenUnconnected=off  PortName=LGData  Element=Nose_WOW
  Out Bus Element4 : Outport  Port=2  VectorParamsAs1DForOutWhenUnconnected=off  PortName=LGData  Element=Nose_GearCmprs
  Out Bus Element5 : Outport  Port=2  VectorParamsAs1DForOutWhenUnconnected=off  PortName=LGData  Element=Nose_LG_down
  Out Bus Element6 : Outport  Port=2  VectorParamsAs1DForOutWhenUnconnected=off  PortName=LGData  Element=LeftMain_WOW
  Out Bus Element7 : Outport  Port=2  VectorParamsAs1DForOutWhenUnconnected=off  PortName=LGData  Element=LeftMain_GearCmprs
  Out Bus Element8 : Outport  Port=2  VectorParamsAs1DForOutWhenUnconnected=off  PortName=LGData  Element=LeftMain_LG_down
  Out Bus Element9 : Outport  Port=2  VectorParamsAs1DForOutWhenUnconnected=off  PortName=LGData  Element=RightMain_WOW
  Out Bus Element10 : Outport  Port=2  VectorParamsAs1DForOutWhenUnconnected=off  PortName=LGData  Element=RightMain_GearCmprs
  Out Bus Element11 : Outport  Port=2  VectorParamsAs1DForOutWhenUnconnected=off  PortName=LGData  Element=RightMain_LG_down
  wires:
  In Bus Element4/1 -> L Main Gear Geometry Forces and Moments/1(ground_z_ft)
  In Bus Element3/1 -> L Main Gear Geometry Forces and Moments/2(plant)
  In Bus Element1/1 -> R Main Gear Geometry Forces and Moments/2(plant)
  In Bus Element2/1 -> Nose Gear Geometry Forces and Moments/2(plant)
  R Main Gear Geometry Forces and Moments/1(FM) -> Sum2/2
  L Main Gear Geometry Forces and Moments/1(FM) -> Sum2/1
  R Main Gear Geometry Forces and Moments/3(GearCmprs) -> Out Bus Element10/1
  R Main Gear Geometry Forces and Moments/2(WOW) -> Out Bus Element9/1
  L Main Gear Geometry Forces and Moments/2(WOW) -> Out Bus Element6/1
  L Main Gear Geometry Forces and Moments/3(GearCmprs) -> Out Bus Element7/1
  RightMain/1 -> R Main Gear Geometry Forces and Moments/3(GearLoc)
  Nose/1 -> Nose Gear Geometry Forces and Moments/3(GearLoc)
  Pos_full_extend_ft Rows are X,Y,Z;cols are Left,Right,Nose gear Measured from CG in fts/1 -> LeftMain/1, Nose/1, RightMain/1
  Nose Gear Geometry Forces and Moments/1(FM) -> Sum2/3
  Nose Gear Geometry Forces and Moments/2(WOW) -> Out Bus Element3/1
  Nose Gear Geometry Forces and Moments/3(GearCmprs) -> Out Bus Element4/1
  Sum2/1 -> FM/1
  LeftMain/1 -> L Main Gear Geometry Forces and Moments/3(GearLoc)
  LG_cmd/1 -> Demux/1
  Demux/1 -> Out Bus Element5/1
  Demux/2 -> Out Bus Element11/1
  Demux/3 -> Out Bus Element8/1
  In Bus Element5/1 -> R Main Gear Geometry Forces and Moments/1(ground_z_ft)
  In Bus Element6/1 -> Nose Gear Geometry Forces and Moments/1(ground_z_ft)

== system Linearize_Bare_Airframe/Vehicle/Propulsion ==
  note: 繞"固定座標旋轉"旋轉(外在旋轉extrinsic rotation)
  note: Thrust Vector Nozzle Module 向量噴嘴模組
  note: Commands_TVC_rY_pitch_deg
      | Commands_TVC_rZ_yaw_deg
      | Commands_TVC_lY_pitch_deg
      | Commands_TVC_lZ_yaw_deg
  note: Inlet 進氣道
  note: 高度限制 0 ~ 50000 ft
      | 馬赫數限制 0 ~ 1 馬赫
  Bus Element In2 : Inport  PortName=fadec_cmd
  In Bus Element3 : Inport  PortName=fadec_cmd  Element=thrust
  In Bus Element1 : Inport  Port=2  PortName=EnvData  Element=Mach
  Bus Element In1 : Inport  Port=3  PortName=PlantData  Element=beta
  Bus Element In : Inport  Port=3  PortName=PlantData  Element=alpha
  In Bus Element : Inport  Port=3  PortName=PlantData  Element=altitude
  Actuators : Subsystem
  Afterburning Turbofan Jet Engine : Subsystem
  Cos : Trigonometry  Operator=cos
  Cos1 : Trigonometry  Operator=cos
  Gain1 : Gain  Gain=0.5
  IC1 : InitialCondition  Commented=through  Value=IC.thrust_lbf
  Product : Product  Inputs=3
  Thrust Vector Nozzle ZY1 : Subsystem
  nozzle position1 : Constant  Value=ac.lt1
  nozzle position2 : Constant  Value=ac.mt
  r2d1 : Gain  Gain=-1  SaturateOnIntegerOverflow=on  OutDataTypeStr=Inherit: Same as input  ParamDataTypeStr=Inherit: Same as input
  FM : Outport
  Bus Element Out : Outport  Port=2  PortName=ActSensor_Out
  Bus Element Out1 : Outport  Port=3  PortName=PropData  Element=Tx
  Bus Element Out2 : Outport  Port=3  PortName=PropData  Element=Ty
  Bus Element Out3 : Outport  Port=3  PortName=PropData  Element=Tz
  Bus Element Out4 : Outport  Port=3  PortName=PropData  Element=T
  Bus Element Out5 : Outport  Port=3  PortName=PropData  Element=engine_state
  wires:
  Actuators/2(ActSensor_Out) -> Bus Element Out/1
  nozzle position1/1 -> Thrust Vector Nozzle ZY1/3(" lt1")
  Actuators/1(ActPositions) -> Thrust Vector Nozzle ZY1/2(Actuator (deg))
  Thrust Vector Nozzle ZY1/1(FM) -> FM/1
  Product/1 -> Afterburning Turbofan Jet Engine/1(Mach)
  r2d1/1 -> Afterburning Turbofan Jet Engine/2(H (ft))
  Cos/1 -> Product/2
  Bus Element In1/1 -> Cos1/1  "beta (rad)"
  In Bus Element1/1 -> Product/1
  Cos1/1 -> Product/3
  Bus Element In/1 -> Cos/1  "alpha (rad)"
  In Bus Element/1 -> r2d1/1
  Bus Element In2/1 -> Actuators/1(Commands)
  Thrust Vector Nozzle ZY1/2(Tx) -> Bus Element Out1/1
  Thrust Vector Nozzle ZY1/3(Ty) -> Bus Element Out2/1
  Thrust Vector Nozzle ZY1/4(Tz) -> Bus Element Out3/1
  nozzle position2/1 -> Thrust Vector Nozzle ZY1/4(" mt")
  IC1/1 -> Gain1/1, Bus Element Out4/1  "thrust"
  Afterburning Turbofan Jet Engine/1(T (lbf)) -> IC1/1  "thrust"
  Afterburning Turbofan Jet Engine/2(engine_state) -> Bus Element Out5/1
  In Bus Element3/1 -> Afterburning Turbofan Jet Engine/3(Tc (lbf))  "Commands_Tc"
  Gain1/1 -> Thrust Vector Nozzle ZY1/1(T1)  "thrust"

== system Linearize_Bare_Airframe/Vehicle/Propulsion(two_nozzles) ==
  note: Thrust Vector Nozzle Module 向量噴嘴模組
  note: Commands_TVC_ry_pitch_deg
      | Commands_TVC_rz_yaw_deg
      | Commands_TVC_ly_pitch_deg
      | Commands_TVC_lz_yaw_deg
  note: Inlet 進氣道
  note: 高度限制 0 ~ 50000 ft
      | 馬赫數限制 0 ~ 1 馬赫
  Bus Element In2 : Inport  PortName=fadec_cmd
  In Bus Element3 : Inport  PortName=fadec_cmd  Element=thrust
  In Bus Element1 : Inport  Port=2  PortName=EnvData  Element=Mach
  Bus Element In1 : Inport  Port=3  PortName=PlantData  Element=beta
  Bus Element In : Inport  Port=3  PortName=PlantData  Element=alpha
  In Bus Element : Inport  Port=3  PortName=PlantData  Element=altitude
  Actuators : Subsystem
  Actuators1 : Subsystem
  Add{,1..5} (6 alike) : Sum
  Afterburning Turbofan Jet Engine : Subsystem
  Bus Creator : BusCreator  Inputs=4
  Cos : Trigonometry  Operator=cos
  Cos1 : Trigonometry  Operator=cos
  Gain1 : Gain  Gain=0.5
  IC1 : InitialCondition  Commented=through  Value=IC.thrust_lbf
  Mux2 : Mux  Inputs=6
  Product : Product  Inputs=3
  Thrust Vector Nozzle ZY1 : Subsystem
  Thrust Vector Nozzle ZY2 : Subsystem
  nozzle position1 : Constant  Value=ac.lt1
  nozzle position2 : Constant  Value=ac.mt
  nozzle position3 : Constant  Value=ac.lt1
  nozzle position4 : Constant  Value=ac.mt
  r2d1 : Gain  Gain=-1  SaturateOnIntegerOverflow=on  OutDataTypeStr=Inherit: Same as input  ParamDataTypeStr=Inherit: Same as input
  FM : Outport
  Bus Element Out : Outport  Port=2  PortName=ActSensor_Out
  Bus Element Out4 : Outport  Port=3  PortName=PropData  Element=T
  Bus Element Out5 : Outport  Port=3  PortName=PropData  Element=engine_state
  Bus Element Out15 : Outport  Port=3  PortName=PropData  Element=Tx
  Bus Element Out16 : Outport  Port=3  PortName=PropData  Element=Ty
  Bus Element Out17 : Outport  Port=3  PortName=PropData  Element=Tz
  wires:
  nozzle position1/1 -> Thrust Vector Nozzle ZY1/3(" lt1")
  Actuators/1(ActPositions) -> Thrust Vector Nozzle ZY1/2(Actuator (deg))
  Product/1 -> Afterburning Turbofan Jet Engine/1(Mach)
  r2d1/1 -> Afterburning Turbofan Jet Engine/2(H (ft))
  Cos/1 -> Product/2
  Bus Element In1/1 -> Cos1/1  "beta (rad)"
  In Bus Element1/1 -> Product/1
  Cos1/1 -> Product/3
  Bus Element In/1 -> Cos/1  "alpha (rad)"
  In Bus Element/1 -> r2d1/1
  Bus Element In2/1 -> Actuators/1(Commands), Actuators1/1(Commands)
  Thrust Vector Nozzle ZY1/1(Trx) -> Add/1
  Thrust Vector Nozzle ZY1/2(Try) -> Add1/1
  Thrust Vector Nozzle ZY1/3(Trz) -> Add2/1
  nozzle position2/1 -> Thrust Vector Nozzle ZY1/4(" mt")
  IC1/1 -> Gain1/1, Bus Element Out4/1  "thrust"
  Afterburning Turbofan Jet Engine/1(T (lbf)) -> IC1/1  "thrust"
  Afterburning Turbofan Jet Engine/2(engine_state) -> Bus Element Out5/1
  In Bus Element3/1 -> Afterburning Turbofan Jet Engine/3(Tc (lbf))  "Commands_Tc"
  Gain1/1 -> Thrust Vector Nozzle ZY1/1(T1), Thrust Vector Nozzle ZY2/1(T1)  "thrust"
  Thrust Vector Nozzle ZY1/4(Mrx) -> Add3/1
  Thrust Vector Nozzle ZY1/5(Mry) -> Add4/1
  Thrust Vector Nozzle ZY1/6(Mrz) -> Add5/1
  nozzle position3/1 -> Thrust Vector Nozzle ZY2/3(" lt1")
  nozzle position4/1 -> Thrust Vector Nozzle ZY2/4(" mt")
  Actuators1/1(ActPositions) -> Thrust Vector Nozzle ZY2/2(Actuator (deg))
  Thrust Vector Nozzle ZY2/1(Tlx) -> Add/2
  Thrust Vector Nozzle ZY2/2(Tly) -> Add1/2
  Thrust Vector Nozzle ZY2/3(Tlz) -> Add2/2
  Thrust Vector Nozzle ZY2/4(Mlx) -> Add3/2
  Thrust Vector Nozzle ZY2/5(Mly) -> Add4/2
  Thrust Vector Nozzle ZY2/6(Mlz) -> Add5/2
  Bus Creator/1 -> Bus Element Out/1
  Add/1 -> Mux2/1, Bus Element Out15/1
  Add1/1 -> Mux2/2, Bus Element Out16/1
  Add2/1 -> Mux2/3, Bus Element Out17/1
  Add3/1 -> Mux2/4
  Add4/1 -> Mux2/5
  Add5/1 -> Mux2/6
  Mux2/1 -> FM/1
  Actuators/2(ActSensor_Out.TVC_ry_pitch_deg) -> Bus Creator/1
  Actuators/3(ActSensor_Out.TVC_rz_yaw_deg) -> Bus Creator/2
  Actuators1/2(ActSensor_Out.TVC_ly_pitch_deg) -> Bus Creator/3
  Actuators1/3(ActSensor_Out.TVC_lz_yaw_deg) -> Bus Creator/4

== system Linearize_Bare_Airframe/Vehicle/6DOF (Quaternion)/Accerlation_offset ==
  note: [eBook]2015 Flight vehicle system identification - a time domain methodology, Second Edition_10.8
  axyz_cg : Inport
  p : Inport  Port=2
  q : Inport  Port=3
  r : Inport  Port=4
  p_dot : Inport  Port=5
  q_dot : Inport  Port=6
  r_dot : Inport  Port=7
  position_x : Inport  Port=8
  position_y : Inport  Port=9
  position_z : Inport  Port=10
  ax_bias : Inport  Port=11
  ay_bias : Inport  Port=12
  az_bias : Inport  Port=13
  Demux : Demux  Outputs=3
  Mux : Mux  Inputs=3
  accerlation_x : Subsystem
  accerlation_y : Subsystem
  accerlation_z : Subsystem
  axyz_offset : Outport
  wires:
  az_bias/1 -> accerlation_z/10(az_bias)
  r/1 -> accerlation_x/3(r), accerlation_y/3(r), accerlation_z/5(r)
  r_dot/1 -> accerlation_y/8(r_dot), accerlation_x/6(r_dot)
  position_z/1 -> accerlation_z/4(position_z), accerlation_y/7(position_z), accerlation_x/9(position_z)
  p/1 -> accerlation_z/2(p), accerlation_y/2(p), accerlation_x/5(p)
  ay_bias/1 -> accerlation_y/10(ay_bias)
  position_y/1 -> accerlation_z/9(position_y), accerlation_y/4(position_y), accerlation_x/7(position_y)
  p_dot/1 -> accerlation_y/6(p_dot), accerlation_z/8(p_dot)
  ax_bias/1 -> accerlation_x/10(ax_bias)
  Demux/3 -> accerlation_z/1(az_cg)  "az_cg"
  position_x/1 -> accerlation_y/9(position_x), accerlation_z/7(position_x), accerlation_x/4(position_x)
  q/1 -> accerlation_x/2(q), accerlation_z/3(q), accerlation_y/5(q)
  accerlation_x/1(ax_as) -> Mux/1
  q_dot/1 -> accerlation_z/6(q_dot), accerlation_x/8(q_dot)
  Demux/2 -> accerlation_y/1(ay_cg)  "ay_cg"
  Demux/1 -> accerlation_x/1(ax_cg)  "ax_cg"
  axyz_cg/1 -> Demux/1
  accerlation_y/1(ay_as) -> Mux/2
  accerlation_z/1(az_as) -> Mux/3
  Mux/1 -> axyz_offset/1

== system Linearize_Bare_Airframe/Vehicle/6DOF (Quaternion)/DCM ==
  note: ${\left[\begin{array}{c} \phi \\ \theta \\ \psi \end{array}\right]}\begin{array}{c} X\\ Y\\ Z \end{array}\to {\left[\begin{array}{c} \psi \\ \theta \\ \phi \end{array}\right]}\begin{array}{c} Z\\ Y\\ X \end{array}$
  note: $Rotation\ Order:ZYX\to \left(\psi ,\theta ,\phi \right)$
  note: ${\left[\begin{array}{c} \phi \\ \theta \\ \psi \end{array}\right]}\begin{array}{c} X\\ Y\\ Z \end{array}$
  note: 慣性座標轉至體座標的旋轉矩陣
  note: 體座標轉至慣性座標的旋轉矩陣
  Euler : Inport
  Rotation Angles to Direction Cosine Matrix : sharedtransform/Rotation Angles to Direction Cosine Matrix  rotationOrder=ZYX  aMode=aMode
      settings: SourceProductBaseCode=AE,PW,DR,MT,VE
  Selector : Selector  InputPortWidth=3  IndexOptions=Index vector (dialog)  Indices=[3 2 1]  OutputSizes=1
  Transpose : Math  Operator=transpose
  DCM_eb : Outport
  DCM_be : Outport  Port=2
  wires:
  Selector/1 -> Rotation Angles to Direction Cosine Matrix/1
  Rotation Angles to Direction Cosine Matrix/1 -> DCM_be/1, Transpose/1
  Transpose/1 -> DCM_eb/1
  Euler/1 -> Selector/1

== system Linearize_Bare_Airframe/Vehicle/Actuators (no roll off)1/Engine block ==
  Mach : Inport
  Attitude : Inport  Port=2
  Add : Sum  Inputs=+-
  Add1 : Sum
  Add2 : Sum
  Constant : Constant
  Constant1 : Constant  Value=0
  Gain : Gain  Gain=64.94
  Gain1 : Gain  Gain=217.38
  If : If  IfExpression=u1<50  ElseIfExpressions=u1>=50  ShowElse=off
  If Action Subsystem : Subsystem  TreatAsAtomicUnit=on
  If Action Subsystem1 : Subsystem  TreatAsAtomicUnit=on
  If Action Subsystem2 : Subsystem  TreatAsAtomicUnit=on
  If Action Subsystem3 : Subsystem  TreatAsAtomicUnit=on
  If1 : If  IfExpression=u1<50  ElseIfExpressions=u1>=50  ShowElse=off
  Mux : Mux  Inputs=2
  Mux1 : Mux  Inputs=2
  Mux4 : Mux  Inputs=5
  Thrust Tidle : Interpolation_n-D  Table=|  InternalRulePriority=Speed
      | [1060	670	880	1140	1500	1860
      | 635	425	690	1010	1330	1700
      | 60	25	345	755	1130	1525
      | -1020	-710	-300	350	910	1360
      | -2700	-1900	-1300	-247	600	1100
      | -3600	-1400	-595	-342	-200	700]
  Thrust Tmax : Interpolation_n-D  Table=reshape([20000,21420,22700,24240,26070,28886,15000,15700,16860,18910,21075,23319,10800,11225,12250,13760,15975,18300,7000,7323,8154,9285,11115,13484,4000,4435,5000,5700,6860,8642,2500,2600,2835,3215,3950,5057],6,6)  InternalRulePriority=Speed
  Thrust Tmil : Interpolation_n-D  Table=|  InternalRulePriority=Speed
      | [12680	9150	6200	3950	2450	1400
      | 12680	9150	6313	4040	2470	1400
      | 12610	9312	6610	4290	2600	1560
      | 12640	9839	7090	4660	2840	1660
      | 12390	10176	7750	5320	3250	1930
      | 11680	9848	8050	6100	3800	2310]
  To Workspace : ToWorkspace  VariableName=T_max_min  SaveFormat=Timeseries  SampleTime=-1
  To Workspace1 : ToWorkspace  VariableName=check_engine  SaveFormat=Timeseries  SampleTime=-1
  To Workspace2 : ToWorkspace  VariableName=Mach_alt_input  SaveFormat=Timeseries  SampleTime=-1
  attitude Prelookup : PreLookup  BreakpointsData=[0,10000,20000,30000,40000,50000]  IndexSearchMethod=Linear search  BeginIndexSearchUsingPreviousIndexResult=on  DiagnosticForOutOfRangeInput=Warning
  constant : Constant  Value=117.38
  mach Prelookup : PreLookup  BreakpointsData=[0,0.2,0.4,0.6,0.8,1]  IndexSearchMethod=Linear search  BeginIndexSearchUsingPreviousIndexResult=on  DiagnosticForOutOfRangeInput=Warning
  T_max : Outport  VectorParamsAs1DForOutWhenUnconnected=off
  T_min : Outport  Port=2  VectorParamsAs1DForOutWhenUnconnected=off
  wires:
  Mach/1 -> Mux/2, mach Prelookup/1
  Attitude/1 -> attitude Prelookup/1, Mux/1
  Add2/1 -> T_min/1, Mux1/2
  Add1/1 -> T_max/1, Mux1/1
  attitude Prelookup/2 -> Thrust Tidle/4, Thrust Tmil/4, Thrust Tmax/4
  Mux1/1 -> To Workspace/1
  Thrust Tmil/1 -> Mux4/4
  Mux/1 -> To Workspace2/1
  Gain1/1 -> Add/1
  If Action Subsystem1/1(T_max1) -> Add1/2
  Constant/1 -> Gain1/1
  mach Prelookup/1 -> Thrust Tidle/1, Thrust Tmil/1, Thrust Tmax/1
  If/2 -> If Action Subsystem1/Action
  If1/2 -> If Action Subsystem3/Action
  If Action Subsystem3/1(T_min) -> Add2/2
  If Action Subsystem2/1(T_min) -> Add2/1
  If1/1 -> If Action Subsystem2/Action
  Gain/1 -> Mux4/2, If1/1
  If Action Subsystem/1(T_max1) -> Add1/1
  Thrust Tmax/1 -> Mux4/5
  mach Prelookup/2 -> Thrust Tidle/2, Thrust Tmil/2, Thrust Tmax/2
  Thrust Tidle/1 -> Mux4/3
  If/1 -> If Action Subsystem/Action
  Add/1 -> Mux4/1, If/1
  constant/1 -> Add/2
  Mux4/1 -> If Action Subsystem1/1("input "), If Action Subsystem2/1("input "), If Action Subsystem3/1("input "), To Workspace1/1, If Action Subsystem/1("input ")
  Constant1/1 -> Gain/1
  attitude Prelookup/1 -> Thrust Tidle/3, Thrust Tmil/3, Thrust Tmax/3
